simulink model "simulacionesP10"  (R2015a)
settings: Solver=ode45  StartTime=0.0  StopTime=10.0  RelTol=1e-3
libraries: fl_lib x54, nesl_utility x20
settings Model: Creator=Jesus  LastModifiedBy=Jesus

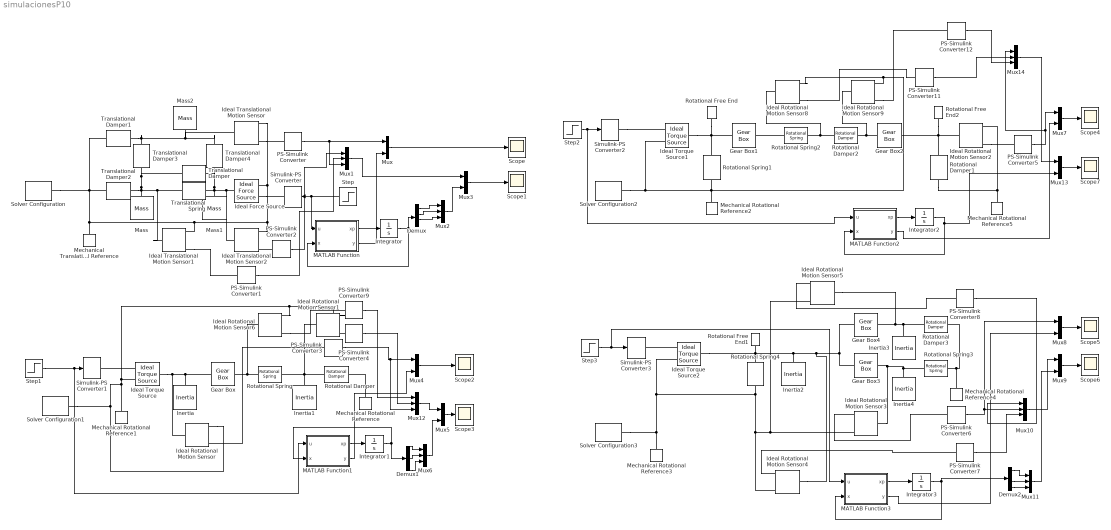
== system simulacionesP10 ==
  Demux : Demux  Outputs=6
  Demux1 : Demux  Outputs=5
  Demux2 : Demux
  Gear Box : fl_lib/Mechanical/Mechanisms/Gear Box  ratio=100/30  t_in_specify=off  t_in_priority=High  t_in=0 N*m  t_out_specify=off  t_out_priority=High  t_out=0 N*m
  Gear Box1 : fl_lib/Mechanical/Mechanisms/Gear Box  ratio=300/30  t_in_specify=off  t_in_priority=High  t_in=0 N*m  t_out_specify=off  t_out_priority=High  t_out=0 N*m
  Gear Box2 : fl_lib/Mechanical/Mechanisms/Gear Box  ratio=100/10  t_in_specify=off  t_in_priority=High  t_in=0 N*m  t_out_specify=off  t_out_priority=High  t_out=0 N*m
  Gear Box3 : fl_lib/Mechanical/Mechanisms/Gear Box  ratio=10  t_in_specify=off  t_in_priority=High  t_in=0 N*m  t_out_specify=off  t_out_priority=High  t_out=0 N*m
  Gear Box4 : fl_lib/Mechanical/Mechanisms/Gear Box  ratio=5  t_in_specify=off  t_in_priority=High  t_in=0 N*m  t_out_specify=off  t_out_priority=High  t_out=0 N*m
  Ideal Force Source : fl_lib/Mechanical/Mechanical Sources/Ideal Force Source
  Ideal Rotational Motion Sensor{,1..6,8..9} (9 alike) : fl_lib/Mechanical/Mechanical Sensors/Ideal Rotational Motion Sensor  offset=0 rad
  Ideal Torque Source : fl_lib/Mechanical/Mechanical Sources/Ideal Torque Source
  Ideal Torque Source1 : fl_lib/Mechanical/Mechanical Sources/Ideal Torque Source
  Ideal Torque Source2 : fl_lib/Mechanical/Mechanical Sources/Ideal Torque Source
  Ideal Translational Motion Sensor : fl_lib/Mechanical/Mechanical Sensors/Ideal Translational Motion Sensor  offset=0 m
  Ideal Translational Motion Sensor1 : fl_lib/Mechanical/Mechanical Sensors/Ideal Translational Motion Sensor  offset=0 m
  Ideal Translational Motion Sensor2 : fl_lib/Mechanical/Mechanical Sensors/Ideal Translational Motion Sensor  offset=0 m
  Inertia : fl_lib/Mechanical/Rotational Elements/Inertia  inertia=50 kg*m^2  w_specify=off  w_priority=High  w=0 rad/s  t_specify=off  t_priority=High  t=0 N*m
  Inertia1 : fl_lib/Mechanical/Rotational Elements/Inertia  inertia=100 kg*m^2  w_specify=off  w_priority=High  w=0 rad/s  t_specify=off  t_priority=High  t=0 N*m
  Inertia2 : fl_lib/Mechanical/Rotational Elements/Inertia  inertia=3 kg*m^2  w_specify=off  w_priority=High  w=0 rad/s  t_specify=off  t_priority=High  t=0 N*m
  Inertia3 : fl_lib/Mechanical/Rotational Elements/Inertia  inertia=200 kg*m^2  w_specify=off  w_priority=High  w=0 rad/s  t_specify=off  t_priority=High  t=0 N*m
  Inertia4 : fl_lib/Mechanical/Rotational Elements/Inertia  inertia=200 kg*m^2  w_specify=off  w_priority=High  w=0 rad/s  t_specify=off  t_priority=High  t=0 N*m
  Integrator : Integrator  InitialCondition=[0 0 0 0 0 0]
  Integrator1 : Integrator  InitialCondition=[0 0 0 0 0]
  Integrator2 : Integrator  InitialCondition=[0 0 0]
  Integrator3 : Integrator  InitialCondition=[0 0 0 0]
  MATLAB Function : MATLAB Function  TreatAsAtomicUnit=on
  MATLAB Function1 : MATLAB Function  TreatAsAtomicUnit=on
  MATLAB Function2 : MATLAB Function  TreatAsAtomicUnit=on
  MATLAB Function3 : MATLAB Function  TreatAsAtomicUnit=on
  Mass : fl_lib/Mechanical/Translational Elements/Mass  mass=2 kg  v_specify=off  v_priority=High  v=0 m/s  f_specify=off  f_priority=High  f=0 N
  Mass1 : fl_lib/Mechanical/Translational Elements/Mass  mass=1 kg  v_specify=off  v_priority=High  v=0 m/s  f_specify=off  f_priority=High  f=0 N
  Mass2 : fl_lib/Mechanical/Translational Elements/Mass  mass=1 kg  v_specify=off  v_priority=High  v=0 m/s  f_specify=off  f_priority=High  f=0 N
  Mechanical Rotational Reference{,1..5} (6 alike) : fl_lib/Mechanical/Rotational Elements/Mechanical Rotational Reference
  Mechanical Translational Reference : fl_lib/Mechanical/Translational Elements/Mechanical Translational Reference
  Mux{,3..5,7..9,13} (8 alike) : Mux  Inputs=2
  Mux{1..2,6,10..12,14} (7 alike) : Mux  Inputs=3
  PS-Simulink Converter{,1..9,11..12} (12 alike) : nesl_utility/PS-Simulink Converter  PhysicalDomain=network_engine_domain  SubClassName=ps_output  LeftPortType=input  RightPortType=output  PseudoPeriodic=off  Frequencies=[]  Unit=1  AffineConversion=off
  Rotational Damper : fl_lib/Mechanical/Rotational Elements/Rotational Damper  D=100 N*m/(rad/s)  w_specify=off  w_priority=High  w=0 rad/s  t_specify=off  t_priority=High  t=0 N*m
  Rotational Damper1 : fl_lib/Mechanical/Rotational Elements/Rotational Damper  D=200 N*m/(rad/s)  w_specify=off  w_priority=High  w=0 rad/s  t_specify=off  t_priority=High  t=0 N*m
  Rotational Damper2 : fl_lib/Mechanical/Rotational Elements/Rotational Damper  D=3 N*m/(rad/s)  w_specify=off  w_priority=High  w=0 rad/s  t_specify=off  t_priority=High  t=0 N*m
  Rotational Damper3 : fl_lib/Mechanical/Rotational Elements/Rotational Damper  D=1000 N*m/(rad/s)  w_specify=off  w_priority=High  w=0 rad/s  t_specify=off  t_priority=High  t=0 N*m
  Rotational Free End : fl_lib/Mechanical/Rotational Elements/Rotational Free End  w_specify=on  w_priority=High  w=0 rad/s
  Rotational Free End1 : fl_lib/Mechanical/Rotational Elements/Rotational Free End  w_specify=off  w_priority=High  w=0 rad/s
  Rotational Free End2 : fl_lib/Mechanical/Rotational Elements/Rotational Free End  w_specify=on  w_priority=High  w=0 rad/s
  Rotational Spring : fl_lib/Mechanical/Rotational Elements/Rotational Spring  spr_rate=100 N*m/rad  w_specify=off  w_priority=High  w=0 rad/s  t_specify=off  t_priority=High  t=0 N*m  phi_specify=off  phi_priority=High  phi=0 rad
  Rotational Spring1 : fl_lib/Mechanical/Rotational Elements/Rotational Spring  spr_rate=1/10 N*m/rad  w_specify=off  w_priority=High  w=0 rad/s  t_specify=off  t_priority=High  t=0 N*m  phi_specify=off  phi_priority=High  phi=0 rad
  Rotational Spring2 : fl_lib/Mechanical/Rotational Elements/Rotational Spring  spr_rate=2 N*m/rad  w_specify=off  w_priority=High  w=0 rad/s  t_specify=off  t_priority=High  t=0 N*m  phi_specify=off  phi_priority=High  phi=0 rad
  Rotational Spring3 : fl_lib/Mechanical/Rotational Elements/Rotational Spring  spr_rate=250 N*m/rad  w_specify=off  w_priority=High  w=0 rad/s  t_specify=off  t_priority=High  t=0 N*m  phi_specify=off  phi_priority=High  phi=0 rad
  Rotational Spring4 : fl_lib/Mechanical/Rotational Elements/Rotational Spring  spr_rate=3 N*m/rad  w_specify=off  w_priority=High  w=0 rad/s  t_specify=off  t_priority=High  t=0 N*m  phi_specify=off  phi_priority=High  phi=0 rad
  Scope{,1..7} (8 alike) : Scope
      Scope settings: YMin=-0.34151  YMax=3.07359
      Scope1 settings: YMin=2.27  YMax=2.48
      Scope2 settings: YMin=2.27  YMax=2.48  SaveName=ScopeData2
      Scope3 settings: YMin=2.27  YMax=2.48  SaveName=ScopeData3
      Scope4 settings: YMin=2.27  YMax=2.48  SaveName=ScopeData4
      Scope5 settings: YMin=0  YMax=0.014  SaveName=ScopeData5
      Scope6 settings: YMin=0  YMax=0.014  SaveName=ScopeData6
      Scope7 settings: YMin=2.27  YMax=2.48  SaveName=ScopeData7
  Simulink-PS Converter{,1..3} (4 alike) : nesl_utility/Simulink-PS Converter  PhysicalDomain=network_engine_domain  SubClassName=ps_input  LeftPortType=input  RightPortType=output  PseudoPeriodic=off  Frequencies=[]  NoiseDistribution=none  NoiseParameters=[]  Unit=1  AffineConversion=off  InputFiltering=off  SimscapeFilterOrder=1  InputFilterTimeConstant=0.001  UdotUserProvided=1
  Solver Configuration : nesl_utility/Solver Configuration  PhysicalDomain=network_engine_domain  SubClassName=solver  LeftPortType=input  RightPortType=generic  Accelerate=off  Tones=[]  Harmonics=[]  SimulateNoise=off  Profile=off  UseLocalSampling=off  EnableSwitchedLinearOptims=on  FrequencyDomain=off  UseCCode=off  RelTol=0.001  AbsTol=1e-06  MinStep=1e-09  ToWorkspace=off  RevertToSquareIcSolve=off  NumHomotopyIterations=100  DoDC=off  ResidualTolerance=1e-09  UseLocalSolver=off  LocalSolverChoice=NE_BACKWARD_EULER_ADVANCER  LocalSolverSampleTime=0.001  DoFixedCost=off  MaxNonlinIter=3  MaxModeIter=2  LinearAlgebra=Sparse  DelaysMemoryBudget=1024  AutomaticFiltering=on  FilteringTimeConstant=0.001
  Solver Configuration1 : nesl_utility/Solver Configuration  PhysicalDomain=network_engine_domain  SubClassName=solver  LeftPortType=input  RightPortType=generic  Accelerate=off  Tones=[]  Harmonics=[]  SimulateNoise=off  Profile=off  UseLocalSampling=off  EnableSwitchedLinearOptims=on  FrequencyDomain=off  UseCCode=off  RelTol=0.001  AbsTol=1e-06  MinStep=1e-09  ToWorkspace=off  RevertToSquareIcSolve=off  NumHomotopyIterations=100  DoDC=off  ResidualTolerance=1e-09  UseLocalSolver=off  LocalSolverChoice=NE_BACKWARD_EULER_ADVANCER  LocalSolverSampleTime=0.001  DoFixedCost=off  MaxNonlinIter=3  MaxModeIter=2  LinearAlgebra=Sparse  DelaysMemoryBudget=1024  AutomaticFiltering=on  FilteringTimeConstant=0.001
  Solver Configuration2 : nesl_utility/Solver Configuration  PhysicalDomain=network_engine_domain  SubClassName=solver  LeftPortType=input  RightPortType=generic  Accelerate=off  Tones=[]  Harmonics=[]  SimulateNoise=off  Profile=off  UseLocalSampling=off  EnableSwitchedLinearOptims=on  FrequencyDomain=off  UseCCode=off  RelTol=0.001  AbsTol=1e-06  MinStep=1e-09  ToWorkspace=off  RevertToSquareIcSolve=off  NumHomotopyIterations=100  DoDC=off  ResidualTolerance=1e-09  UseLocalSolver=on  LocalSolverChoice=NE_BACKWARD_EULER_ADVANCER  LocalSolverSampleTime=0.001  DoFixedCost=on  MaxNonlinIter=3  MaxModeIter=2  LinearAlgebra=Sparse  DelaysMemoryBudget=1024  AutomaticFiltering=on  FilteringTimeConstant=0.001
  Solver Configuration3 : nesl_utility/Solver Configuration  PhysicalDomain=network_engine_domain  SubClassName=solver  LeftPortType=input  RightPortType=generic  Accelerate=off  Tones=[]  Harmonics=[]  SimulateNoise=off  Profile=off  UseLocalSampling=off  EnableSwitchedLinearOptims=on  FrequencyDomain=off  UseCCode=off  RelTol=0.001  AbsTol=1e-06  MinStep=1e-09  ToWorkspace=off  RevertToSquareIcSolve=off  NumHomotopyIterations=100  DoDC=off  ResidualTolerance=1e-09  UseLocalSolver=off  LocalSolverChoice=NE_BACKWARD_EULER_ADVANCER  LocalSolverSampleTime=0.001  DoFixedCost=off  MaxNonlinIter=3  MaxModeIter=2  LinearAlgebra=Sparse  DelaysMemoryBudget=1024  AutomaticFiltering=on  FilteringTimeConstant=0.001
  Step{,1..3} (4 alike) : Step  SampleTime=0
  Translational Damper{,1..4} (5 alike) : fl_lib/Mechanical/Translational Elements/Translational Damper  D=1 N/(m/s)  v_specify=off  v_priority=High  v=0 m/s  f_specify=off  f_priority=High  f=0 N
  Translational Spring : fl_lib/Mechanical/Translational Elements/Translational Spring  spr_rate=2 N/m  v_specify=off  v_priority=High  v=0 m/s  f_specify=off  f_priority=High  f=0 N  x_specify=off  x_priority=High  x=0 m
  wires:
  Step/1 -> MATLAB Function/1(u), Simulink-PS Converter/1
  MATLAB Function/1(xp) -> Integrator/1
  Integrator/1 -> MATLAB Function/2(x), Demux/1
  Mux/1 -> Scope/1
  PS-Simulink Converter/1 -> Mux1/3, Mux/1
  MATLAB Function/2(y) -> Mux/2
  PS-Simulink Converter2/1 -> Mux1/1
  PS-Simulink Converter1/1 -> Mux1/2
  Mux1/1 -> Mux3/1
  Demux/1 -> Mux2/1
  Demux/3 -> Mux2/2
  Demux/5 -> Mux2/3
  Mux2/1 -> Mux3/2
  Mux3/1 -> Scope1/1
  Step1/1 -> MATLAB Function1/1(u), Simulink-PS Converter1/1
  MATLAB Function1/1(xp) -> Integrator1/1
  Mux4/1 -> Scope2/1
  PS-Simulink Converter3/1 -> Mux12/3, Mux4/1
  MATLAB Function1/2(y) -> Mux4/2
  Mux5/1 -> Scope3/1
  Integrator1/1 -> MATLAB Function1/2(x), Demux1/1
  Demux1/1 -> Mux6/1
  Demux1/3 -> Mux6/2
  Mux6/1 -> Mux5/2
  MATLAB Function2/1(xp) -> Integrator2/1
  Integrator2/1 -> Mux13/2, MATLAB Function2/2(x)
  Step3/1 -> MATLAB Function3/1(u), Simulink-PS Converter3/1
  MATLAB Function3/1(xp) -> Integrator3/1
  Integrator3/1 -> MATLAB Function3/2(x), Demux2/1
  PS-Simulink Converter5/1 -> Mux14/1, Mux7/1
  Step2/1 -> Simulink-PS Converter2/1, MATLAB Function2/1(u)
  Mux7/1 -> Scope4/1
  MATLAB Function2/2(y) -> Mux7/2
  Mux8/1 -> Scope5/1
  MATLAB Function3/2(y) -> Mux8/2
  PS-Simulink Converter6/1 -> Mux10/2, Mux8/1
  Mux9/1 -> Scope6/1
  PS-Simulink Converter8/1 -> Mux10/1
  PS-Simulink Converter7/1 -> Mux10/3
  Mux10/1 -> Mux9/1
  Mux11/1 -> Mux9/2
  Demux2/4 -> Mux11/3
  Demux2/3 -> Mux11/2
  Demux2/1 -> Mux11/1
  Demux1/5 -> Mux6/3
  PS-Simulink Converter9/1 -> Mux12/1
  PS-Simulink Converter4/1 -> Mux12/2
  Mux12/1 -> Mux5/1
  Mux13/1 -> Scope7/1
  PS-Simulink Converter11/1 -> Mux14/2
  PS-Simulink Converter12/1 -> Mux14/3
  Mux14/1 -> Mux13/1
  connections:
  Ideal Force Source/LConn1 -- Translational Damper/RConn1 -- Translational Damper4/RConn1 -- Mass1/LConn1 -- Translational Spring/RConn1 -- Ideal Translational Motion Sensor2/LConn1
  Translational Damper1/RConn1 -- Ideal Translational Motion Sensor/LConn1 -- Translational Damper4/LConn1 -- Mass2/LConn1 -- Translational Damper3/LConn1
  Ideal Translational Motion Sensor/RConn1 -- Ideal Translational Motion Sensor2/RConn1 -- Mechanical Translational Reference/LConn1 -- Solver Configuration/RConn1 -- Translational Damper1/LConn1 -- Translational Damper2/LConn1 -- Ideal Translational Motion Sensor1/RConn1 -- Ideal Force Source/RConn2
  Ideal Force Source/RConn1 -- Simulink-PS Converter/RConn1
  Ideal Translational Motion Sensor/RConn3 -- PS-Simulink Converter/LConn1
  Translational Damper2/RConn1 -- Translational Damper/LConn1 -- Translational Damper3/RConn1 -- Mass/LConn1 -- Ideal Translational Motion Sensor1/LConn1 -- Translational Spring/LConn1
  Ideal Translational Motion Sensor1/RConn3 -- PS-Simulink Converter1/LConn1
  PS-Simulink Converter2/LConn1 -- Ideal Translational Motion Sensor2/RConn3
  Gear Box/LConn1 -- Ideal Torque Source/LConn1 -- Ideal Rotational Motion Sensor/LConn1 -- Inertia/LConn1
  Rotational Spring/LConn1 -- Gear Box/RConn1 -- Ideal Rotational Motion Sensor6/LConn1
  Inertia1/LConn1 -- Rotational Spring/RConn1 -- Ideal Rotational Motion Sensor1/LConn1 -- Rotational Damper/LConn1
  Mechanical Rotational Reference/LConn1 -- Rotational Damper/RConn1
  Ideal Torque Source/RConn1 -- Simulink-PS Converter1/RConn1
  Mechanical Rotational Reference1/LConn1 -- Solver Configuration1/RConn1 -- Ideal Rotational Motion Sensor/RConn1 -- Ideal Rotational Motion Sensor6/RConn1 -- Ideal Rotational Motion Sensor1/RConn1 -- Ideal Torque Source/RConn2
  PS-Simulink Converter3/LConn1 -- Ideal Rotational Motion Sensor/RConn3
  PS-Simulink Converter4/LConn1 -- Ideal Rotational Motion Sensor1/RConn3
  Ideal Torque Source2/RConn1 -- Simulink-PS Converter3/RConn1
  Mechanical Rotational Reference3/LConn1 -- Solver Configuration3/RConn1 -- Ideal Rotational Motion Sensor5/RConn1 -- Ideal Rotational Motion Sensor3/RConn1 -- Ideal Rotational Motion Sensor4/RConn1 -- Rotational Spring4/RConn1 -- Ideal Torque Source2/RConn2
  Ideal Torque Source2/LConn1 -- Rotational Free End1/LConn1 -- Rotational Spring4/LConn1 -- Ideal Rotational Motion Sensor4/LConn1 -- Gear Box4/LConn1 -- Gear Box3/LConn1 -- Inertia2/LConn1
  Rotational Damper3/LConn1 -- Inertia3/LConn1 -- Ideal Rotational Motion Sensor5/LConn1 -- Gear Box4/RConn1
  Rotational Spring3/LConn1 -- Ideal Rotational Motion Sensor3/LConn1 -- Gear Box3/RConn1 -- Inertia4/LConn1
  Mechanical Rotational Reference4/LConn1 -- Rotational Damper3/RConn1 -- Rotational Spring3/RConn1
  Ideal Rotational Motion Sensor3/RConn3 -- PS-Simulink Converter6/LConn1
  Rotational Spring1/LConn1 -- Rotational Free End/LConn1 -- Gear Box1/LConn1 -- Ideal Torque Source1/LConn1
  Mechanical Rotational Reference2/LConn1 -- Ideal Rotational Motion Sensor8/RConn1 -- Ideal Rotational Motion Sensor9/RConn1 -- Ideal Torque Source1/RConn2 -- Solver Configuration2/RConn1 -- Rotational Spring1/RConn1
  Rotational Spring2/LConn1 -- Gear Box1/RConn1
  Rotational Damper2/LConn1 -- Ideal Rotational Motion Sensor8/LConn1 -- Rotational Spring2/RConn1
  Gear Box2/LConn1 -- Ideal Rotational Motion Sensor9/LConn1 -- Rotational Damper2/RConn1
  Rotational Damper1/LConn1 -- Rotational Free End2/LConn1 -- Ideal Rotational Motion Sensor2/LConn1 -- Gear Box2/RConn1
  Simulink-PS Converter2/RConn1 -- Ideal Torque Source1/RConn1
  Ideal Rotational Motion Sensor2/RConn3 -- PS-Simulink Converter5/LConn1
  PS-Simulink Converter7/LConn1 -- Ideal Rotational Motion Sensor4/RConn3
  Ideal Rotational Motion Sensor5/RConn3 -- PS-Simulink Converter8/LConn1
  Rotational Damper1/RConn1 -- Mechanical Rotational Reference5/LConn1 -- Ideal Rotational Motion Sensor2/RConn1
  Ideal Rotational Motion Sensor6/RConn3 -- PS-Simulink Converter9/LConn1
  Ideal Rotational Motion Sensor8/RConn3 -- PS-Simulink Converter11/LConn1
  Ideal Rotational Motion Sensor9/RConn3 -- PS-Simulink Converter12/LConn1

== matlab function simulacionesP10/MATLAB Function1 ==
  data: xp output; u input; y output; x input
function [xp,y] = fcn(u,x)
%#codegen
A=[0 1 0 0 0;-9/50 0 3/5 0 0;0 0 0 1 0;3/10 0 -1 -1 0;0 3/10 0 0 0];
B=[0 1/50 0 0 0]';
C=[1 0 0 0 0];
xp=A*x+B*u;
y = C*x;

== matlab function simulacionesP10/MATLAB Function ==
  data: xp output; u input; y output; x input
function [xp,y] = fcn(u,x)
%#codegen
A=[0 1 0 0 0 0;-1 -3/2 1 1/2 0 1/2;0 0 0 1 0 0;2 1 -2 -2 0 1;0 0 0 0 0 1;0 1 0 1 0 -3];
B=[0 0 0 1 0 0]';
C=[0 0 0 0 1 0];
xp=A*x+B*u;
y = C*x;

== matlab function simulacionesP10/MATLAB Function2 ==
  data: xp output; u input; y output; x input
function [xp,y] = fcn(u,x)
%#codegen
A=[-25/18 0 0;-5/6 0 0;-1/12 0 0];
B=[25/18 5/6 1/12]';
C=[0 0 1];
xp=A*x+B*u;
y = C*x;

== matlab function simulacionesP10/MATLAB Function3 ==
  data: xp output; u input; y output; x input
function [xp,y] = fcn(u,x)
%#codegen
A=[0 1 0 0;-11/26 -40/13 0 0;0 1/10 0 0;0 1/5 0 0];
B=[0 1/13 0 0]';
C=[0 0 1 0];
xp=A*x+B*u;
y = C*x;
